simulink model "simulation_commande_sliding_mode_2_fuzzy"  (R2020a)
settings: Solver=VariableStepAuto  StartTime=0.0  StopTime=100  RelTol=1e-3
values from neighbouring files (symbols this model uses):
  a = 1    [Adap.m]    (also in Adaptive_control_Non_linear.m = 2; HOSM.m; projet_AAV.m; sys.m)
  b = 2    [Adaptive_Control_Linear.m]    (also in Adaptive_control_Non_linear.m; HOSM.m = 1; feedback-integrator.m = 3; mini_projet.m = 3)
  lambda = 0.3    [fuzzy.m]    (also in projet_AAV.m = 1)
settings Model: Creator=lenovo  LastModifiedBy=lenovo
settings SolverCC: ZeroCrossAlgorithm=Adaptive
settings DebuggingCC: IgnoredZcDiagnostic=none

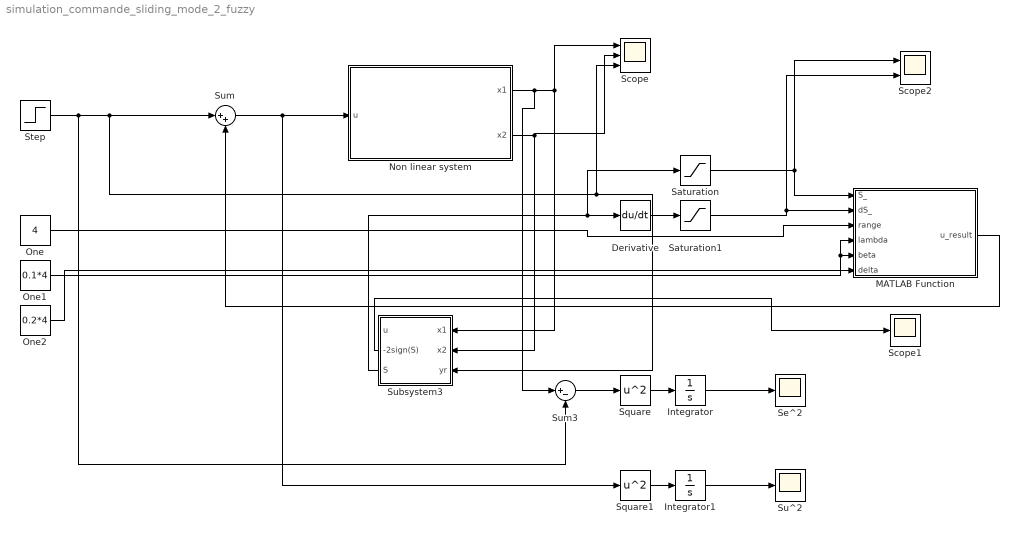
== system simulation_commande_sliding_mode_2_fuzzy ==
  Derivative : Derivative
  Integrator : Integrator
  Integrator1 : Integrator
  MATLAB Function : MATLAB Function  TreatAsAtomicUnit=on
  Non linear system : Subsystem
  One : Constant  Value=4  OutDataTypeStr=Inherit: Inherit via back propagation
  One1 : Constant  Value=0.1*4  OutDataTypeStr=Inherit: Inherit via back propagation
  One2 : Constant  Value=0.2*4  OutDataTypeStr=Inherit: Inherit via back propagation
  Saturation : Saturate  UpperLimit=4  LowerLimit=-4
  Saturation1 : Saturate  UpperLimit=4  LowerLimit=-4
  Scope : Scope  NumInputPorts=3
  Scope1 : Scope
  Scope2 : Scope  NumInputPorts=2
  Se^2 : Scope
  Square : Math  Operator=square  SaturateOnIntegerOverflow=on
  Square1 : Math  Operator=square  SaturateOnIntegerOverflow=on
  Step : Step  Time=0  SampleTime=0
  Su^2 : Scope
  Subsystem3 : Subsystem
  Sum : Sum  Inputs=|++
  Sum3 : Sum  Inputs=|+-
  wires:
  Sum/1 -> Square1/1, Non linear system/1(u)
  Non linear system/2(x2) -> Scope/2, Subsystem3/2(x2)
  Subsystem3/2(-2sign(S)) -> Scope1/1
  Sum3/1 -> Square/1
  Square/1 -> Integrator/1
  Integrator/1 -> Se^2/1
  Step/1 -> Sum3/2, Subsystem3/3(yr), Scope/3, Sum/1
  Integrator1/1 -> Su^2/1
  Square1/1 -> Integrator1/1
  Non linear system/1(x1) -> Sum3/1, Subsystem3/1(x1), Scope/1
  One/1 -> MATLAB Function/3(range)
  One1/1 -> MATLAB Function/5(beta), MATLAB Function/4(lambda)
  One2/1 -> MATLAB Function/6(delta)
  MATLAB Function/1(u_result) -> Sum/2
  Subsystem3/3(S) -> Saturation/1, Derivative/1
  Derivative/1 -> Saturation1/1
  Saturation/1 -> MATLAB Function/1(S_), Scope2/1
  Saturation1/1 -> Scope2/2, MATLAB Function/2(dS_)

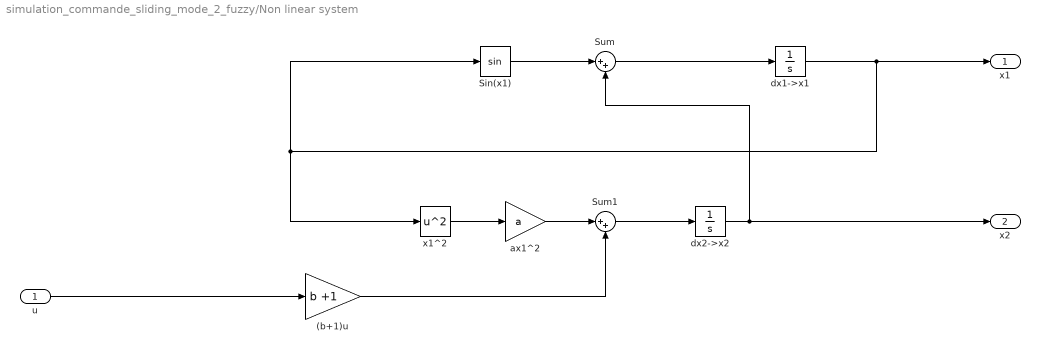
== system simulation_commande_sliding_mode_2_fuzzy/Non linear system ==
  u : Inport
  (b+1)u : Gain  Gain=b +1
  Sin(x1) : Trigonometry
  Sum : Sum  Inputs=|++
  Sum1 : Sum  Inputs=|++
  ax1^2 : Gain  Gain=a
  dx1->x1 : Integrator
  dx2->x2 : Integrator
  x1^2 : Math  Operator=square  SaturateOnIntegerOverflow=on
  x1 : Outport
  x2 : Outport  Port=2
  wires:
  (b+1)u/1 -> Sum1/2
  dx2->x2/1 -> x2/1, Sum/2
  u/1 -> (b+1)u/1
  ax1^2/1 -> Sum1/1
  dx1->x1/1 -> Sin(x1)/1, x1^2/1, x1/1
  Sin(x1)/1 -> Sum/1
  x1^2/1 -> ax1^2/1
  Sum1/1 -> dx2->x2/1
  Sum/1 -> dx1->x1/1

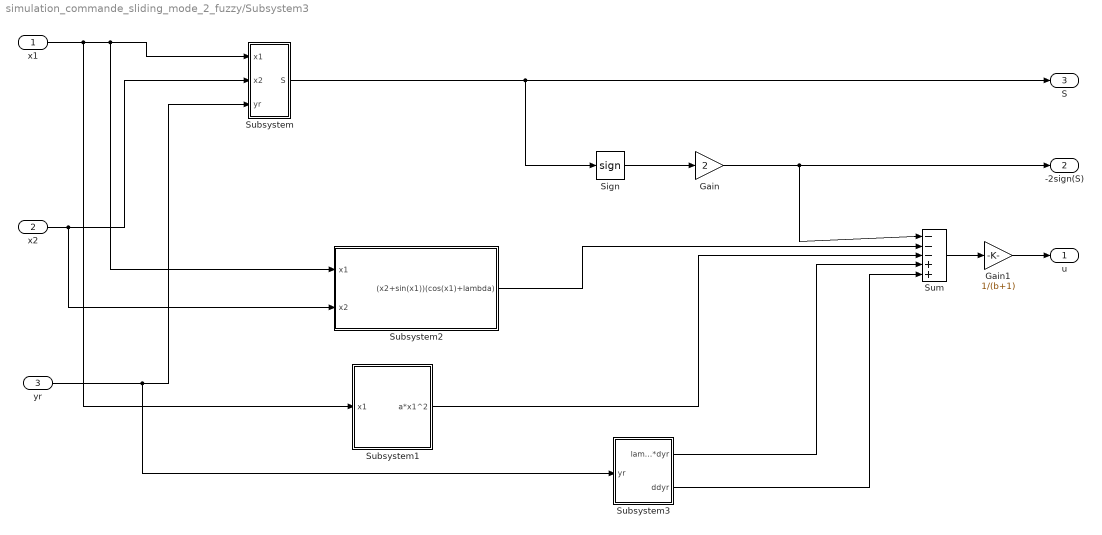
== system simulation_commande_sliding_mode_2_fuzzy/Subsystem3 ==
  x1 : Inport
  x2 : Inport  Port=2
  yr : Inport  Port=3
  Gain : Gain  Gain=2
  Gain1 : Gain  Gain=1/(b+1)
  Sign : Signum
  Subsystem : Subsystem
  Subsystem1 : Subsystem
  Subsystem2 : Subsystem
  Subsystem3 : Subsystem
  Sum : Sum  Inputs=|---++
  u : Outport
  -2sign(S) : Outport  Port=2
  S : Outport  Port=3
  wires:
  Gain/1 -> -2sign(S)/1, Sum/1
  Sum/1 -> Gain1/1
  Sign/1 -> Gain/1
  Subsystem2/1((x2+sin(x1))(cos(x1)+lambda)) -> Sum/2
  Gain1/1 -> u/1
  Subsystem1/1(a*x1^2) -> Sum/3
  Subsystem3/1(lambda*dyr) -> Sum/4
  x1/1 -> Subsystem1/1("x1 "), Subsystem2/1("x1 "), Subsystem/1(x1)
  x2/1 -> Subsystem2/2(x2), Subsystem/2(x2)
  yr/1 -> Subsystem3/1(yr), Subsystem/3(yr)
  Subsystem/1(S) -> S/1, Sign/1
  Subsystem3/2(ddyr) -> Sum/5

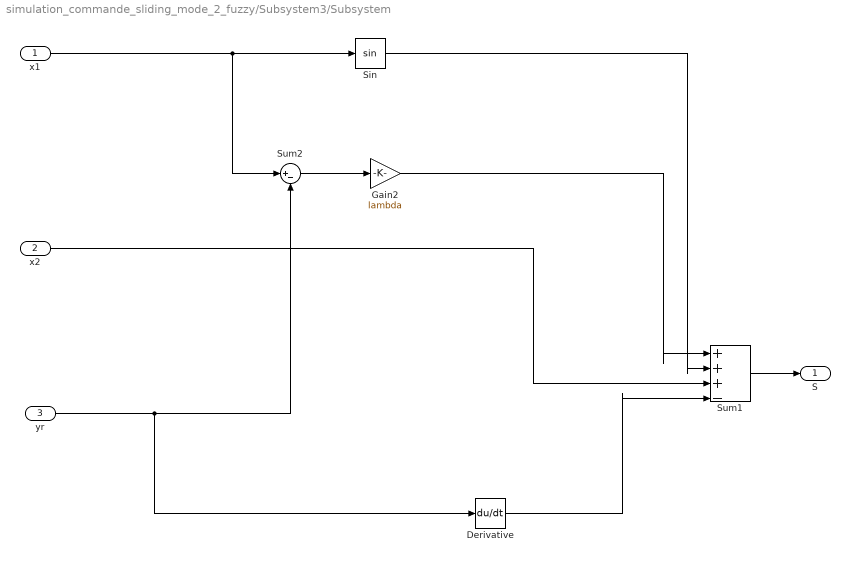
== system simulation_commande_sliding_mode_2_fuzzy/Subsystem3/Subsystem ==
  x1 : Inport
  x2 : Inport  Port=2
  yr : Inport  Port=3
  Derivative : Derivative
  Gain2 : Gain  Gain=lambda
  Sin : Trigonometry
  Sum1 : Sum  Inputs=|+++-
  Sum2 : Sum  Inputs=|+-
  S : Outport
  wires:
  x1/1 -> Sum2/1, Sin/1
  x2/1 -> Sum1/3
  Gain2/1 -> Sum1/1
  yr/1 -> Derivative/1, Sum2/2
  Sin/1 -> Sum1/2
  Sum2/1 -> Gain2/1
  Derivative/1 -> Sum1/4
  Sum1/1 -> S/1

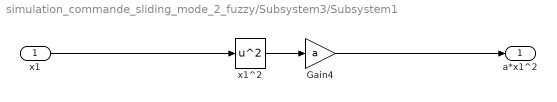
== system simulation_commande_sliding_mode_2_fuzzy/Subsystem3/Subsystem1 ==
  "x1 " : Inport
  Gain4 : Gain  Gain=a
  x1^2 : Math  Operator=square  SaturateOnIntegerOverflow=on
  a*x1^2 : Outport
  wires:
  x1^2/1 -> Gain4/1
  Gain4/1 -> a*x1^2/1
  "x1 "/1 -> x1^2/1

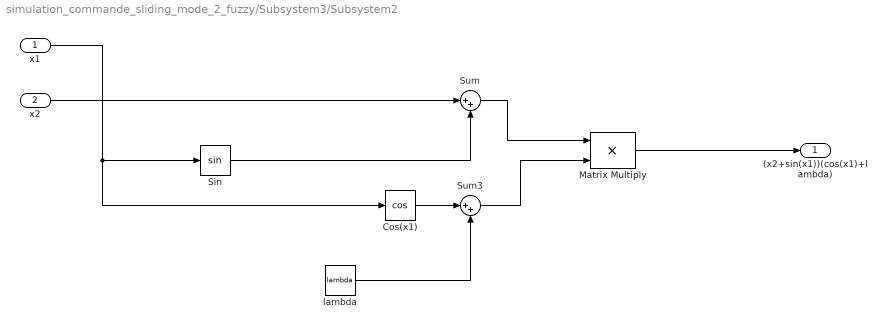
== system simulation_commande_sliding_mode_2_fuzzy/Subsystem3/Subsystem2 ==
  "x1 " : Inport
  x2 : Inport  Port=2
  Cos(x1) : Trigonometry  Operator=cos
  Matrix Multiply : Product
  Sin : Trigonometry
  Sum : Sum  Inputs=|++
  Sum3 : Sum  Inputs=|++
  lambda : Constant  Value=lambda  OutDataTypeStr=Inherit: Inherit via back propagation
  (x2+sin(x1))(cos(x1)+lambda) : Outport
  wires:
  Cos(x1)/1 -> Sum3/1
  lambda/1 -> Sum3/2
  x2/1 -> Sum/1
  Matrix Multiply/1 -> (x2+sin(x1))(cos(x1)+lambda)/1
  Sum/1 -> Matrix Multiply/1
  Sum3/1 -> Matrix Multiply/2
  "x1 "/1 -> Cos(x1)/1, Sin/1
  Sin/1 -> Sum/2

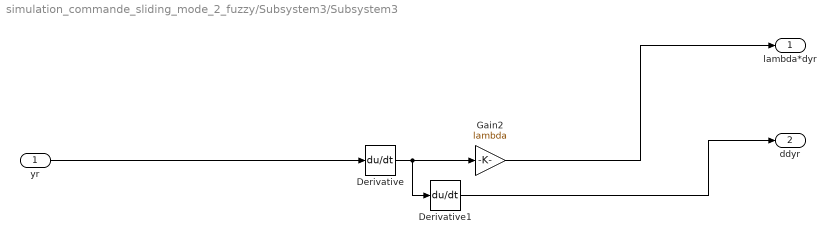
== system simulation_commande_sliding_mode_2_fuzzy/Subsystem3/Subsystem3 ==
  yr : Inport
  Derivative : Derivative
  Derivative1 : Derivative
  Gain2 : Gain  Gain=lambda
  lambda*dyr : Outport
  ddyr : Outport  Port=2
  wires:
  Derivative/1 -> Derivative1/1, Gain2/1
  Derivative1/1 -> ddyr/1
  yr/1 -> Derivative/1
  Gain2/1 -> lambda*dyr/1

== matlab function simulation_commande_sliding_mode_2_fuzzy/MATLAB Function ==
  data: S_ input; u_result output; dS_ input; range input; lambda input; beta input; delta input
function u_result = fuzzy(S_, dS_, range, lambda, beta , delta)
%% Fuzzy input
% input S
step = 0.01
S = -range:step:range;


Sp = 1/lambda*S;
Sp(S >= lambda ) = 1;
Sp(S <= 0 ) = 0;

Sn = -1/lambda*S;
Sn(S <= -lambda ) = 1;
Sn(S >= 0 ) = 0;

S0 = -1/lambda*abs(S) + 1;
S0(S <= -lambda ) = 0;
S0(S >= lambda ) = 0;

 
% input dS
dS = -range:step:range;

dSp = 1/beta*dS;
dSp(dS >= beta ) = 1;
dSp(dS <= 0 ) = 0;

dSn = -1/beta*dS;
dSn(dS <= -beta ) = 1;
dSn(dS >= 0 ) = 0;

dS0 = -1/beta*abs(dS) + 1;
dS0(dS <= -beta ) = 0;
dS0(dS >= beta ) = 0;

% Fuzzy output

u = -range:step:range;

up = 1/delta*u;
up(u >= delta ) = 1;
up(u <= 0 ) = 0;

un = -1/delta*u;
un(u <= -delta ) = 1;
un(u >= 0 ) = 0;

u0 = -1/delta*abs(u) + 1;
u0(u <= -delta ) = 0;
u0(u >= delta ) = 0;

% Rules 

it_S = fix(S_/ step) + range/step +1
it_dS = fix(dS_/ step) + range/step +1

% R1 si S>0 et dS> 0 alors u = un
alpha1 = Sp(it_S)*dSp(it_dS);
% R2 si S>0 et dS< 0 alors u = u0
alpha2 = Sp(it_S)*dSn(it_dS);
% R3 si S>0 et dS= 0 alors u = un
alpha3 = Sp(it_S)*dS0(it_dS);

% R4 si S=0 et dS> 0 alors u = un
alpha4 = S0(it_S)*dSp(it_dS);
% R5 si S=0 et dS< 0 alors u = up
alpha5 = S0(it_S)*dSn(it_dS);
% R6 si S=0 et dS= 0 alors u = u0
alpha6 = S0(it_S)*dS0(it_dS);

% R7 si S<0 et dS> 0 alors u = u0
alpha7 = Sn(it_S)*dSp(it_dS);
% R8 si S<0 et dS< 0 alors u = up
alpha8 = Sn(it_S)*dSn(it_dS);
% R9 si S<0 et dS= 0 alors u = up
alpha9 = Sn(it_S)*dS0(it_dS);


ufinal = ((alpha7+ alpha8 + alpha9)*up + (alpha4 + alpha5 + alpha6)*u0 + (alpha1+ alpha2+ alpha3)*un);

sumalpha = (alpha1+ alpha2 + alpha3 + alpha4 + alpha5 + alpha6 + alpha7+ alpha9 +alpha9);

ufinal = ufinal/sumalpha;
ufinal = sum(u.*ufinal)/sum(abs(u))

u_result = ufinal
